simulink model "ls_reg"  (R2017a)
settings: Solver=FixedStepAuto  StartTime=0.0  StopTime=tEnd  FixedStep=dt  RelTol=1e-3
undefined symbols (not defined in the file or in its folder): Ts
libraries: slident x2
settings Model: Creator=e_anderlini  LastModifiedBy=e_anderlini

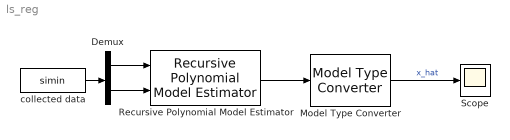
== system ls_reg ==
  Demux : Demux  Outputs=[4,8]
  Model Type Converter : slident/Estimators/Model Type Converter  InputModelType=ARX
      settings: SourceProductName=System Identification Toolbox  SourceProductBaseCode=ID
  Recursive Polynomial Model Estimator : slident/Estimators/Recursive Polynomial Model Estimator  ModelStructure=ARX  InitialEstimateSource=Internal  A0=Aq  B0=Bq  C0=1  D0=1  F0=1  nk=1  P0=1  EstimationMethod=Kalman Filter  AdaptationParameter=0.01  NormalizationBias=eps  OutputError=off  OutputP=off  AddEnablePort=off  Ts=Ts
      settings: SourceProductName=System Identification Toolbox  SourceProductBaseCode=ID
  Scope : Scope
  collected data : FromWorkspace  VariableName=simin  SampleTime=0
  wires:
  Model Type Converter/1 -> Scope/1  "x_hat"
  collected data/1 -> Demux/1
  Demux/2 -> Recursive Polynomial Model Estimator/2
  Demux/1 -> Recursive Polynomial Model Estimator/1
  Recursive Polynomial Model Estimator/1 -> Model Type Converter/1
